simulink model "dynamic_controller_system"  (R2013a)
settings: Solver=ode45  StartTime=0.0  StopTime=250  FixedStep=0.1  RelTol=2e-3
libraries: simulink x5, Controllers x5, DiffSteer_model x2
settings Model: Creator=Felipe  LastModifiedBy=Felipe
settings DataIOCC: MaxDataPoints=10000
settings DebuggingCC: SolverPrmCheckMsg=none

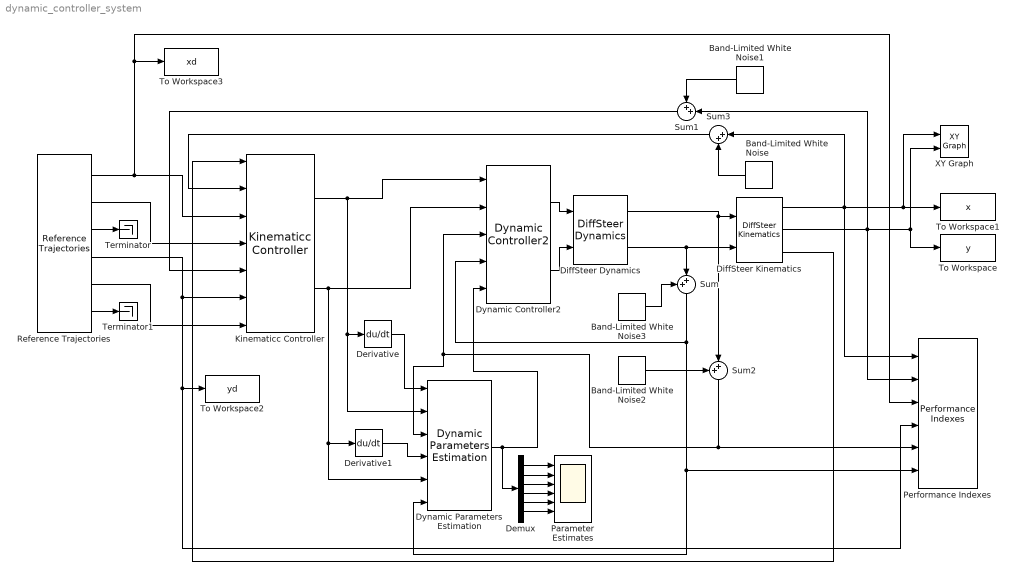
== system dynamic_controller_system ==
  Band-Limited White Noise : simulink/Sources/Band-Limited White Noise  Cov=[0.00002]  Ts=0.1  seed=[23341]
  Band-Limited White Noise1 : simulink/Sources/Band-Limited White Noise  Cov=[0.00002]  Ts=0.1  seed=[20001]
  Band-Limited White Noise2 : simulink/Sources/Band-Limited White Noise  Cov=[0.00005]  Ts=0.1  seed=[11141]
  Band-Limited White Noise3 : simulink/Sources/Band-Limited White Noise  Cov=[0.00005]  Ts=0.1  seed=[01234]
  Demux : Demux  Outputs=6
  Derivative : Derivative
  Derivative1 : Derivative
  DiffSteer Dynamics : DiffSteer_model/DiffSteer Dynamics  umax=0.75  wmax=1.745  dumax=0.3  dwmax=1.745  param=[0.2604 0.2509 -0.000499 0.9965 0.00263 1.0768]
  DiffSteer Kinematics : DiffSteer_model/DiffSteer Kinematics  x0=[-0.5, -0.5, pi]  a=0.2  umax=0.75  wmax=1.745  dumax=0.3  dwmax=1.745
  Dynamic Parameters Estimation : Controllers/Dynamic Parameters Estimation  ku=4  kw=4  lu=1  lw=1  inicia_adapt=50  theta=[0.30822 0.16922 -0.00058 0.80630 -0.00244 1.13994]  gamma=[1.7 1.1 0.5 0.5 0.5 0.5]  sig_mod=[0.01 0.05 0.01 0.01 0.01 0.01]
  Dynamic Controller2 : Controllers/Dynamic  Controller2  ku=4  kw=4  lu=1  lw=1
  Kinematicc Controller : Controllers/Kinematicc Controller  kx=5  ky=5  lx=5  ly=5  a=0.2
  Parameter Estimates : Scope  NumInputPorts=6
      settings: TimeRange=250  YMin=0~0~-1~0~-0.5~0  YMax=10~15~0~6~1~10
  Performance Indexes : Controllers/Performance  Indexes
  Reference Trajectories : Controllers/Reference Trajectories  trajectory_type=2  wf=0.1  raio_ref_1=1  delta_raio=-0.1  t_delta_raio=60  xd=[1, -2]
  Sum : Sum  Inputs=++|
  Sum1 : Sum  Inputs=++|
  Sum2 : Sum  Inputs=++|
  Sum3 : Sum  Inputs=|++
  Terminator : Terminator
  Terminator1 : Terminator
  To Workspace : ToWorkspace  VariableName=y  SampleTime=-1
  To Workspace1 : ToWorkspace  VariableName=x  SampleTime=-1
  To Workspace2 : ToWorkspace  VariableName=yd  SampleTime=-1
  To Workspace3 : ToWorkspace  VariableName=xd  SampleTime=-1
  XY Graph : simulink/Sinks/XY Graph  xmin=-2  xmax=2  ymin=-3  ymax=1  st=-1
  wires:
  Reference Trajectories/1 -> Performance Indexes/3, To Workspace3/1, Kinematicc Controller/3
  Reference Trajectories/2 -> Kinematicc Controller/4
  Reference Trajectories/4 -> Performance Indexes/4, To Workspace2/1, Kinematicc Controller/6
  Reference Trajectories/5 -> Kinematicc Controller/7
  DiffSteer Kinematics/1 -> Sum3/1, XY Graph/1, To Workspace1/1, Performance Indexes/1
  DiffSteer Kinematics/2 -> Sum1/2, XY Graph/2, To Workspace/1, Performance Indexes/2
  DiffSteer Kinematics/3 -> Kinematicc Controller/1
  Dynamic Parameters Estimation/1 -> Demux/1, Dynamic Controller2/5
  Dynamic Controller2/1 -> DiffSteer Dynamics/1
  Dynamic Controller2/2 -> DiffSteer Dynamics/2
  Kinematicc Controller/1 -> Derivative/1, Dynamic Parameters Estimation/2, Dynamic Controller2/1
  Kinematicc Controller/2 -> Derivative1/1, Dynamic Parameters Estimation/5, Dynamic Controller2/2
  Derivative/1 -> Dynamic Parameters Estimation/1
  Derivative1/1 -> Dynamic Parameters Estimation/4
  Reference Trajectories/3 -> Terminator/1
  Reference Trajectories/6 -> Terminator1/1
  DiffSteer Dynamics/2 -> Sum/2, DiffSteer Kinematics/2
  Band-Limited White Noise3/1 -> Sum/1
  Sum/1 -> Dynamic Controller2/4, Dynamic Parameters Estimation/6, Performance Indexes/6
  DiffSteer Dynamics/1 -> Sum2/2, DiffSteer Kinematics/1
  Band-Limited White Noise2/1 -> Sum2/1
  Sum2/1 -> Performance Indexes/5, Dynamic Controller2/3, Dynamic Parameters Estimation/3
  Band-Limited White Noise1/1 -> Sum1/1
  Band-Limited White Noise/1 -> Sum3/2
  Sum3/1 -> Kinematicc Controller/2
  Sum1/1 -> Kinematicc Controller/5
  Demux/6 -> Parameter Estimates/6
  Demux/5 -> Parameter Estimates/5
  Demux/4 -> Parameter Estimates/4
  Demux/3 -> Parameter Estimates/3
  Demux/2 -> Parameter Estimates/2
  Demux/1 -> Parameter Estimates/1
